simulink model "NTCM_TEST_HARNESS_MiLvsSiL"  (R2021a)
settings: Solver=FixedStepAuto  StartTime=0.0  StopTime=End_Time  FixedStep=Sample_Time  RelTol=1e-3  EnableMultiTasking=on
undefined symbols (not defined in the file): GNSScarrierFrequency
settings Model: OrderedModelArguments=off  Creator=zurnmar  LastModifiedBy=zurnmar
settings DataIOCC: ReturnWorkspaceOutputs=off  SignalLoggingName=logsout_new
settings OptimizationCC: UseDivisionForNetSlopeComputation=on  UseFloatMulNetSlope=on  UseSpecifiedMinMax=on  PassReuseOutputArgsAs=Individual arguments  ZeroExternalMemoryAtStartup=off  ZeroInternalMemoryAtStartup=off  EfficientFloat2IntCast=on  LifeSpan=2  EfficientTunableParamExpr=on
settings DebuggingCC: ParameterTunabilityLossMsg=error  AssertControl=DisableAll  SFMachineParentedDataDiag=warning
settings HardwareCC: ProdBitPerPointer=32  ProdBitPerSizeT=32  ProdBitPerPtrDiffT=32  ProdLargestAtomicInteger=LongLong  ProdLargestAtomicFloat=Double  ProdEndianess=BigEndian  ProdWordSize=32  ProdLongLongMode=on  ProdHWDeviceType=Custom Processor->Custom
settings ModelReferenceCC: ModelReferenceNumInstancesAllowed=Single
settings SFSimCC: MATLABDynamicMemAlloc=off
settings RTWCC: SystemTargetFile=ert.tlc  TemplateMakefile=ert_default_tmf  GenerateReport=on  Toolchain=MinGW64 | gmake (64-bit Windows)  BuildConfiguration=Faster Runs  IncludeHyperlinkInReport=on  LaunchReport=on  PortableWordSizes=on  CodeExecutionProfiling=on  CodeProfilingInstrumentation=detailed  GenerateTraceInfo=on  GenerateTraceReport=on  GenerateTraceReportSl=on  GenerateTraceReportSf=on  GenerateTraceReportEml=on  GenerateCodeMetricsReport=on
settings CodeAppCC: ForceParamTrailComments=on  IgnoreCustomStorageClasses=off  MaxIdLength=51  OperatorAnnotations=on  SimulinkDataObjDesc=on  SFDataObjDesc=on  MATLABFcnDesc=on  CustomSymbolStrFcn=$M$F  CustomSymbolStrFcnArg=$N$M  InsertBlockDesc=on  StateflowObjectComments=on  MATLABSourceComments=on  ReqsInCode=on
settings ERTTargetCC: TargetLangStandard=C99 (ISO)  UtilityFuncGeneration=Shared location  GenerateSampleERTMain=on  CombineSignalStateStructs=on  SuppressErrorStatus=on  CodeInterfacePackaging=Reusable function  SupportNonFinite=off  SupportComplex=off  RemoveResetFunc=off  ParenthesesLevel=Maximum  CastingMode=Standards  RootIOFormat=Structure reference  ERTSrcFileBannerTemplate=Myert_code_template.cgt  ERTHdrFileBannerTemplate=Myert_code_template.cgt  ERTDataSrcFileTemplate=Myert_code_template.cgt  ERTDataHdrFileTemplate=Myert_code_template.cgt  ERTCustomFileTemplate=example_file_process.tlc  EnableSignedLeftShifts=off  EnableSignedRightShifts=off

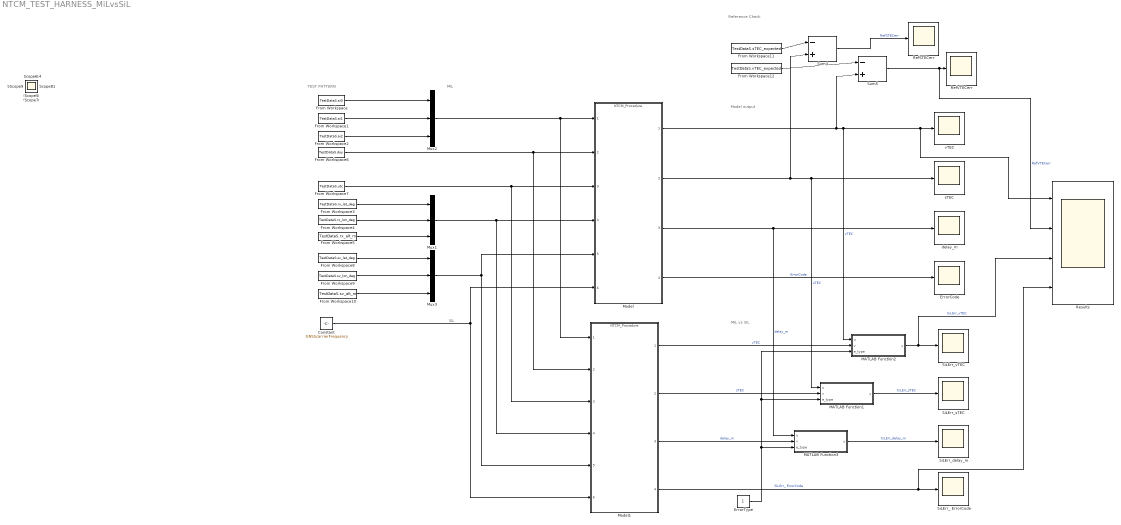
== system NTCM_TEST_HARNESS_MiLvsSiL ==
  note: MIL
  note: Reference Check
  note: Model output
  note: MIL vs SIL
  note: SIL
  note: TEST PATTERN
  Constant : Constant  Value=GNSScarrierFrequency
  ErrorCode : Scope
  ErrorType : Constant
  From Workspace : FromWorkspace  VariableName=TestDataS.ai0  SampleTime=-1  Interpolate=off  OutputAfterFinalValue=Holding final value
  From Workspace1 : FromWorkspace  VariableName=TestDataS.ai1  SampleTime=-1  Interpolate=off  OutputAfterFinalValue=Holding final value
  From Workspace10 : FromWorkspace  VariableName=TestDataS.sv_alt_m  SampleTime=-1  OutputAfterFinalValue=Holding final value
  From Workspace11 : FromWorkspace  VariableName=TestDataS.sTEC_expected  SampleTime=-1
  From Workspace12 : FromWorkspace  VariableName=TestDataS.vTEC_expected  SampleTime=-1
  From Workspace2 : FromWorkspace  VariableName=TestDataS.ai2  SampleTime=-1  Interpolate=off  OutputAfterFinalValue=Holding final value
  From Workspace3 : FromWorkspace  VariableName=TestDataS.rx_lat_deg  SampleTime=-1  Interpolate=off  OutputAfterFinalValue=Holding final value
  From Workspace4 : FromWorkspace  VariableName=TestDataS.rx_lon_deg  SampleTime=-1  Interpolate=off  OutputAfterFinalValue=Holding final value
  From Workspace5 : FromWorkspace  VariableName=TestDataS.rx_alt_m  SampleTime=-1  Interpolate=off  OutputAfterFinalValue=Holding final value
  From Workspace6 : FromWorkspace  VariableName=TestDataS.doy  SampleTime=-1  Interpolate=off  OutputAfterFinalValue=Holding final value
  From Workspace7 : FromWorkspace  VariableName=TestDataS.utc  SampleTime=-1  Interpolate=off  OutputAfterFinalValue=Holding final value
  From Workspace8 : FromWorkspace  VariableName=TestDataS.sv_lat_deg  SampleTime=-1  Interpolate=off  OutputAfterFinalValue=Holding final value
  From Workspace9 : FromWorkspace  VariableName=TestDataS.sv_lon_deg  SampleTime=-1  Interpolate=off  OutputAfterFinalValue=Holding final value
  MATLAB Function1 : MATLAB Function  TreatAsAtomicUnit=on
  MATLAB Function2 : MATLAB Function  TreatAsAtomicUnit=on
  MATLAB Function3 : MATLAB Function  TreatAsAtomicUnit=on
  Model : ModelReference  Description=|  ModelNameDialog=NTCM_Procedure.slx  SimulationMode=Normal  ModelReferenceVersion=1.0
      | /*==========================================================
      |  * NTCM_Procedure_Core.c 
      |  * Implementation of the Galileo NeQuick G ionospheric model. 
      |  * 
      |  *
      |  *
      |  *
      |  *
      |  * INPUT:
      |  * ------
      |  * AzPara		=> alpha0, alpha1, and alpha2 Iono Parameters broadcasted by Galileo
      |  * Doy     		=> Day of the year 
      |  * UTC 			=> UTC Time in hours (0 for midnight)
      |  * llhRecDeg   	=> User position in Longitude[rad], Latitude[rad], height[m] 
      |  * llhSatDeg   	=> Satellite position in Longitude[rad], Latitude[rad], height[m]  
      |  * fcarr      	=> Carrier frequency
      |  *
      |  * Output:
      |  * ------
      |  * vTEC			=> Vertical TEC
      |  * sTEC			=> Slant TEC
      |  * delay_m		=> Signal propagation time delay in [m]
      |  * ErrorCode	=> Error Code (optional)
      |  *
      |  * External parameters:
      |  * ------
      |  * ErrCodeEl                      2U                        /
      |  * ErrCodeIn                      1U                        
      |  * ErrCodeOut                     3U                        
      |  * IPP_RefAltitude                450000.0                  /
      |  * LTd                            14.0                      
      |  * NoErr                          0U                                                                                                                                                                                                                                                                            
      |  * Pf1                            0.4                       
      |  * doy_DAV                        18.0                      
      |  * doy_DSAV                       6.0                                       
      |  * lamGNP_deg                     -71.78                    
      |  * phiGNP_deg                     79.74                     
      |  * phi_c1                         16.0                      
      |  * phi_c2                         -10.0                     
      |  * sigma_c1                       12.0                      
      |  * sigma_c2                       13.0 
      |  * k1                             0.92519                   
      |  * k10                            1.20556                   
      |  * k11                            1.41808                   
      |  * k12                            0.13985                   
      |  * k2                             0.16951                   
      |  * k3                             0.00443                   
      |  * k4                             0.06626                   
      |  * k5                             0.00899                   
      |  * k6                             0.21289                   
      |  * k7                             -0.15414                  
      |  * k8                             -0.38439                  
      |  * k9                             1.14023    
      |  *========================================================*/
  Model1 : ModelReference  ModelNameDialog=NTCM_Procedure.slx  SimulationMode=Software-in-the-loop (SIL)  ModelReferenceVersion=1.0
  Mux1 : Mux  Inputs=3
  Mux2 : Mux  Inputs=3
  Mux3 : Mux  Inputs=3
  RefSTECerr : Scope
  RefVTECerr : Scope
  Results : Scope  NumInputPorts=4
  SiLErr_ ErrorCode : Scope
  SiLErr_delay_m : Scope
  SiLErr_sTEC : Scope
  SiLErr_vTEC : Scope
  Sum4 : Sum  Inputs=|-+
  Sum5 : Sum  Inputs=|-+
  delay_m : Scope
  sTEC : Scope
  vTEC : Scope
  Scope{,1..14} (15 alike) : Scope
  wires:
  Constant/1 -> Model1/6, Model/6
  From Workspace6/1 -> Model1/2, Model/2
  Sum4/1 -> RefSTECerr/1  "RefSTECerr"
  From Workspace8/1 -> Mux3/1
  Model1/2 -> MATLAB Function1/2(v)  "sTEC"
  From Workspace/1 -> Mux2/1
  Mux1/1 -> Model1/4, Model/4
  From Workspace4/1 -> Mux1/2
  Mux3/1 -> Model1/5, Model/5
  From Workspace11/1 -> Sum4/1
  MATLAB Function3/1(y) -> SiLErr_delay_m/1  "SiLErr_delay_m"
  Model1/3 -> MATLAB Function3/2(v)  "delay_m"
  Model/1 -> MATLAB Function2/1(u), Results/1, vTEC/1, Sum5/2  "vTEC"
  From Workspace9/1 -> Mux3/2
  Model/3 -> MATLAB Function3/1(u), delay_m/1  "delay_m"
  From Workspace10/1 -> Mux3/3
  From Workspace2/1 -> Mux2/3
  From Workspace1/1 -> Mux2/2
  From Workspace5/1 -> Mux1/3
  MATLAB Function1/1(y) -> SiLErr_sTEC/1  "SiLErr_sTEC"
  From Workspace3/1 -> Mux1/1
  Mux2/1 -> Model1/1, Model/1
  Model1/1 -> MATLAB Function2/2(v)  "vTEC"
  Model/2 -> MATLAB Function1/1(u), sTEC/1, Sum4/2  "sTEC"
  Model1/4 -> Results/4, SiLErr_ ErrorCode/1  "SiLErr_ ErrorCode"
  Model/4 -> ErrorCode/1  "ErrorCode"
  Sum5/1 -> Results/2, RefVTECerr/1  "RefVTECerr"
  From Workspace12/1 -> Sum5/1
  From Workspace7/1 -> Model1/3, Model/3
  ErrorType/1 -> MATLAB Function3/3(e_type), MATLAB Function2/3(e_type), MATLAB Function1/3(e_type)
  MATLAB Function2/1(y) -> Results/3, SiLErr_vTEC/1  "SiLErr_vTEC"

== matlab function NTCM_TEST_HARNESS_MiLvsSiL/MATLAB Function2 ==
  data: u input; y output; v input; e_type input
function y = Error(u,v,e_type)
% u expected
% v measured
switch e_type
    case 0
        y = abs(v-u);
    case 1
        y = abs(1-v/u);
    case 2
        y= 100*abs(1-v/u);
    otherwise
        y=v-u;
end

== matlab function NTCM_TEST_HARNESS_MiLvsSiL/MATLAB Function3 ==
  data: u input; y output; v input; e_type input
function y = Error(u,v,e_type)
% u expected
% v measured
switch e_type
    case 0
        y = abs(v-u);
    case 1
        y = abs(1-v/u);
    case 2
        y= 100*abs(1-v/u);
    otherwise
        y=v-u;
end

== matlab function NTCM_TEST_HARNESS_MiLvsSiL/MATLAB Function1 ==
  data: u input; y output; v input; e_type input
function y = Error(u,v,e_type)
% u expected
% v measured
switch e_type
    case 0
        y = abs(v-u);
    case 1
        y = abs(1-v/u);
    case 2
        y= 100*abs(1-v/u);
    otherwise
        y=v-u;
end
